simulink model "P2p2"  (R2014a)
settings: Solver=ode1  StartTime=0.0  StopTime=inf  FixedStep=0.002  RelTol=1e-3
PostLoadFcn:
  | qc_set_target_type(getConfigSet(bdroot, 'QUARC Default Target Configuration'));
values from neighbouring files (symbols this model uses):
  K_pd = -2*real(eig)*J_p/L1    [P2_init.m]
  K_pp = abs(eig)^2*J_p/L1    [P2_init.m]
  K_rp = -1.5    [P2_init.m]
undefined symbols (not defined in the file or in its folder): elevation_offset, HIL, Joystick_gain_x, Joystick_gain_y, qc_get_step_size, Vs_star_meas
libraries: simulink_extras x7, quarc_library x7
settings Model: SimulationMode=external  ExtModeTrigDuration=500000  Creator=Rchan  LastModifiedBy=rendellc
settings SolverCC: PositivePriorityOrder=on
settings DataIOCC: SignalLoggingSaveFormat=ModelDataLogs
settings OptimizationCC: ExpressionDepthLimit=2147483647  InitFltsAndDblsToZero=on
settings DebuggingCC: SaveWithParameterizedLinksMsg=none  UnderspecifiedInitializationDetection=Classic  MultiTaskDSMMsg=warning  MultiTaskCondExecSysMsg=none  FcnCallInpInsideContextMsg=UseLocalSettings  StateNameClashWarn=warning
settings RTWCC: SystemTargetFile=quarc_win64.tlc  TemplateMakefile=quarc_default_tmf  Description=QUARC Win64 Target  ProcessScript=quarc_win64_make_rtw_hook
settings STFCustomTargetCC: CPPClassGenCompliant=on
settings GRTTargetCC: ParMdlRefBuildCompliant=off  CompOptLevelCompliant=off  CombineOutputUpdateFcns=off  MatFileLogging=off  GRTInterface=on  ExtMode=on  ExtModeMexFile=quarc_comm

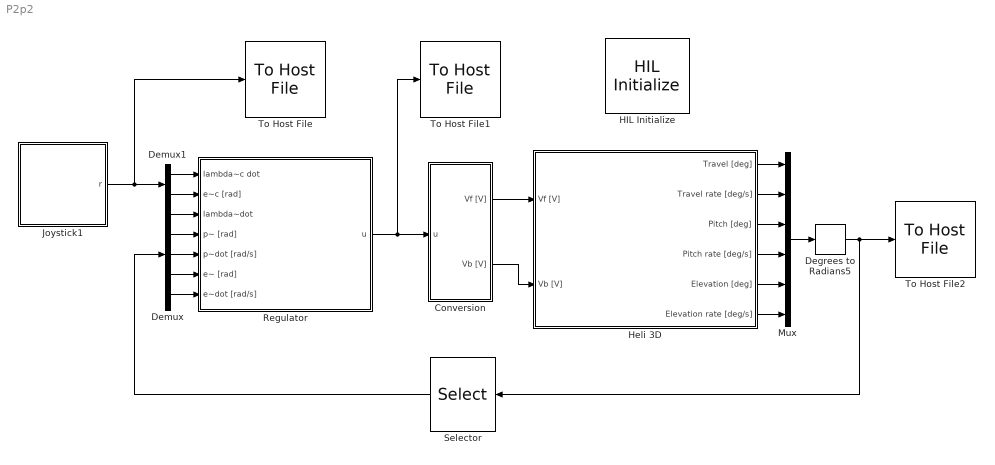
== system P2p2 ==
  Conversion : Subsystem
  Degrees to Radians5 : simulink_extras/Transformations/Degrees to Radians
  Demux : Demux  Outputs=5
  Demux1 : Demux  Outputs=2
  HIL Initialize : quarc_library/Data Acquisition/Generic/Configuration/HIL Initialize  Priority=-99  object_name=HIL-1  board_type=q8_usb  board_number=0  board_options=update_rate=normal;decimation=1  exclusive=off  active=off  hardware_clocks=[0:2]  clock_modes=[]  initial_clock_frequencies=[]  set_clock_params_at_start=off  set_clock_params_at_switch_in=off  set_clock_frequencies_at_start=off  set_clock_frequencies_at_switch_in=off  analog_input_channels=[0:7]  analog_input_maximums=10  analog_input_minimums=-10  set_analog_input_params_at_start=on  set_analog_input_params_at_switch_in=off  analog_output_channels=[0:7]  analog_output_maximums=10  analog_output_minimums=-10  initial_analog_outputs=[0]  final_analog_outputs=[0]  watchdog_analog_outputs=0  set_analog_output_params_at_start=on  set_analog_output_params_at_switch_in=off  set_analog_outputs_at_start=on  set_analog_outputs_at_switch_in=off  set_analog_outputs_at_terminate=on  set_analog_outputs_at_switch_out=off  set_analog_outputs_on_watchdog=off  digital_input_channels=[]  digital_output_channels=[]  digital_output_configuration=[]  initial_digital_outputs=[1]  final_digital_outputs=[1]  watchdog_digital_outputs=[1]  set_digital_output_params_at_start=off  set_digital_output_params_at_switch_in=off  set_digital_outputs_at_start=on  set_digital_outputs_at_switch_in=off  set_digital_outputs_at_terminate=on  set_digital_outputs_at_switch_out=off  set_digital_outputs_on_watchdog=off  encoder_channels=[0:7]  quadrature=[4]  encoder_filter_frequency=[]  initial_encoder_counts=[0]  set_encoder_params_at_start=on  set_encoder_params_at_switch_in=off  set_encoder_counts_at_start=on  set_encoder_counts_at_switch_in=off  pwm_channels=[0:7]  pwm_modes=0  pwm_frequency=99.532799999999995e6/4095  pwm_configuration=[0]  pwm_alignment=[0]  pwm_polarity=[1]  pwm_leading_deadband=[0]  pwm_trailing_deadband=[0]  initial_pwm_outputs=[0]  final_pwm_outputs=[0]  watchdog_pwm_outputs=[0]  set_pwm_params_at_start=on  set_pwm_params_at_switch_in=off  set_pwm_outputs_at_start=on  set_pwm_outputs_at_switch_in=off  set_pwm_outputs_at_terminate=on  set_pwm_outputs_at_switch_out=off  set_pwm_outputs_on_watchdog=off  other_output_channels=[]  initial_other_outputs=[]  final_other_outputs=[]  watchdog_other_outputs=[]  set_other_outputs_at_start=off  set_other_outputs_at_switch_in=off  set_other_outputs_at_terminate=off  set_other_outputs_at_switch_out=off  set_other_outputs_on_watchdog=off
  Heli 3D : Subsystem
  Joystick1 : Subsystem
      mask Display: image('../Common/joy_img.png');
  Mux : Mux  Inputs=6
  Regulator : Subsystem
  Selector : Selector  InputPortWidth=6  Indices=[2 3 4 5 6]
  To Host File : quarc_library/Sinks/To Host/To Host File  file_name=..\..\data\Part 2\P2p2_ref.mat  variable_name=ref  decimation=1  sample_time=-1  file_format=MAT-file v.4  options=No header or footer  append=off  final_file_name=..\..\data\Part 2\P2p2_ref.mat
  To Host File1 : quarc_library/Sinks/To Host/To Host File  file_name=P2p2_u.mat  variable_name=u  decimation=1  sample_time=-1  file_format=MAT-file v.4  options=No header or footer  append=off  final_file_name=P2p2_u.mat
  To Host File2 : quarc_library/Sinks/To Host/To Host File  file_name=P2p2_plant.mat  variable_name=plant  decimation=1  sample_time=-1  file_format=MAT-file v.4  options=No header or footer  append=off  final_file_name=P2p2_plant.mat
  wires:
  Conversion/2(Vb [V]) -> Heli 3D/2(Vb [V])
  Conversion/1(Vf [V]) -> Heli 3D/1(Vf [V])
  Heli 3D/1(Travel [deg]) -> Mux/1
  Heli 3D/2(Travel rate [deg/s]) -> Mux/2
  Heli 3D/3(Pitch [deg]) -> Mux/3
  Heli 3D/4(Pitch rate [deg/s]) -> Mux/4
  Heli 3D/6(Elevation rate [deg/s]) -> Mux/6
  Heli 3D/5(Elevation [deg]) -> Mux/5
  Mux/1 -> Degrees to Radians5/1
  Selector/1 -> Demux/1
  Demux/1 -> Regulator/3(lambda~dot)
  Demux/2 -> Regulator/4(p~ [rad])
  Demux/3 -> Regulator/5("p~dot [rad/s] ")
  Demux/4 -> Regulator/6(e~ [rad])
  Demux/5 -> Regulator/7(e~dot [rad/s])
  Demux1/1 -> Regulator/1(lambda~c dot)
  Demux1/2 -> Regulator/2(e~c [rad])
  Degrees to Radians5/1 -> To Host File2/1, Selector/1
  Joystick1/1(r) -> To Host File/1, Demux1/1
  Regulator/1(u) -> To Host File1/1, Conversion/1(u)

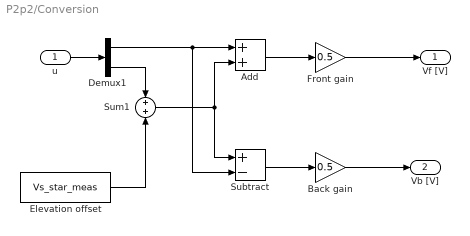
== system P2p2/Conversion ==
  u : Inport
  Add : Sum
  Back gain : Gain  Gain=0.5
  Demux1 : Demux  Outputs=2
  Elevation offset : Constant  Value=Vs_star_meas
  Front gain : Gain  Gain=0.5
  Subtract : Sum  Inputs=+-
  Sum1 : Sum  Inputs=+|+
  Vf [V] : Outport
  Vb [V] : Outport  Port=2
  wires:
  Demux1/1 -> Subtract/2, Add/1
  Subtract/1 -> Back gain/1
  Back gain/1 -> Vb [V]/1
  Add/1 -> Front gain/1
  Front gain/1 -> Vf [V]/1
  Elevation offset/1 -> Sum1/2
  Demux1/2 -> Sum1/1
  Sum1/1 -> Subtract/1, Add/2
  u/1 -> Demux1/1

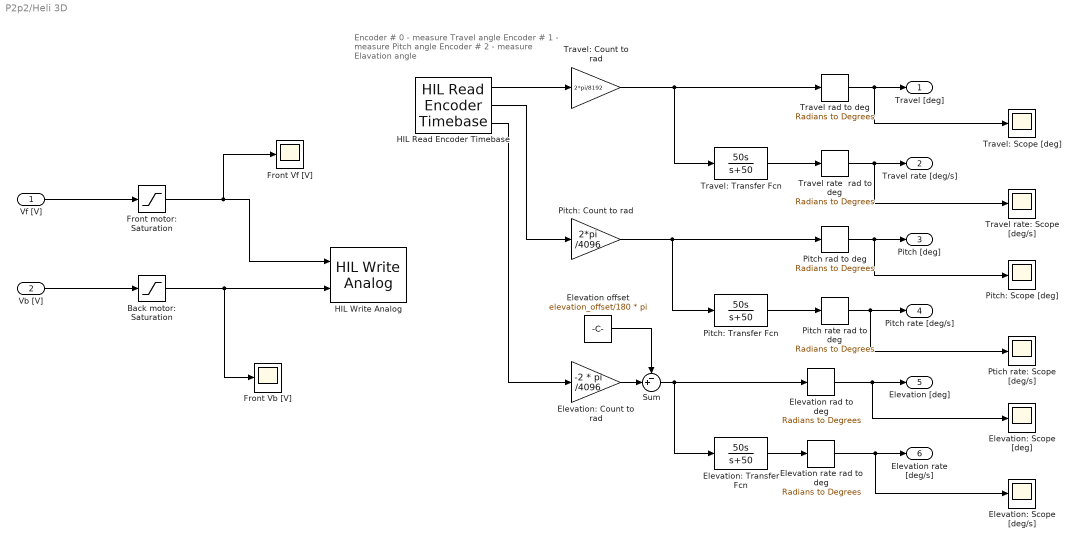
== system P2p2/Heli 3D ==
  note: Encoder # 0 - measure Travel angle
      | Encoder # 1 - measure Pitch angle
      | Encoder # 2 - measure Elavation angle
  Vf [V] : Inport
  Vb [V] : Inport  Port=2
  Back motor: Saturation : Saturate  UpperLimit=5  LowerLimit=-5
  Elevation offset : Constant  Value=elevation_offset/180 * pi
  Elevation rad to deg : simulink_extras/Transformations/Radians to Degrees
  Elevation rate rad to deg : simulink_extras/Transformations/Radians to Degrees
  Elevation: Count to rad : Gain  Gain=-2 * pi /4096
  Elevation: Scope [deg/s] : Scope
      settings: YMin=-15  YMax=15  SaveName=ScopeData13
  Elevation: Scope [deg] : Scope
      settings: YMax=45  SaveName=ScopeData12
  Elevation: Transfer Fcn : TransferFcn  Numerator=[50 0]  Denominator=[1 50]
  Front Vb [V] : Scope
      settings: YMin=-2  SaveName=ScopeData2
  Front Vf [V] : Scope
      settings: YMin=-2
  Front motor: Saturation : Saturate  UpperLimit=5  LowerLimit=-5
  HIL Read Encoder Timebase : quarc_library/Data Acquisition/Generic/Timebases/HIL Read Encoder Timebase  object_name=HIL-1  clock=0  channels=[0:2]  samples_in_buffer=max(ceil(1/qc_get_step_size), 1)  active=on  vector_output=off  data_type_mode=Inherit via back propagation  data_type=double
  HIL Write Analog : quarc_library/Data Acquisition/Generic/Immediate I//O/HIL Write Analog  object_name=HIL-1  channels=[0:1]  sample_time=-1  active=off  vector_input=off
  Pitch rad to deg : simulink_extras/Transformations/Radians to Degrees
  Pitch rate rad to deg : simulink_extras/Transformations/Radians to Degrees
  Pitch: Count to rad : Gain  Gain=2*pi /4096
  Pitch: Scope [deg] : Scope
      settings: YMin=-80  YMax=80  SaveName=ScopeData10
  Pitch: Transfer Fcn : TransferFcn  Numerator=[50 0]  Denominator=[1 50]
  Ptich rate: Scope [deg/s] : Scope
      settings: YMin=-15  YMax=15  SaveName=ScopeData11
  Sum : Sum  Inputs=-+|
  Travel rad to deg : simulink_extras/Transformations/Radians to Degrees
  Travel rate  rad to deg : simulink_extras/Transformations/Radians to Degrees
  Travel rate: Scope [deg/s] : Scope
      settings: YMin=-30  YMax=70  SaveName=ScopeData9
  Travel: Count to rad : Gain  Gain=2*pi/8192
  Travel: Scope [deg] : Scope
      settings: YMin=-250  YMax=2250  SaveName=ScopeData8
  Travel: Transfer Fcn : TransferFcn  Numerator=[50 0]  Denominator=[1 50]
  Travel [deg] : Outport
  Travel rate [deg/s] : Outport  Port=2
  Pitch [deg] : Outport  Port=3
  Pitch rate [deg/s] : Outport  Port=4
  Elevation [deg] : Outport  Port=5
  Elevation rate [deg/s] : Outport  Port=6
  wires:
  HIL Read Encoder Timebase/1 -> Travel: Count to rad/1
  HIL Read Encoder Timebase/2 -> Pitch: Count to rad/1
  HIL Read Encoder Timebase/3 -> Elevation: Count to rad/1
  Travel: Count to rad/1 -> Travel: Transfer Fcn/1, Travel rad to deg/1
  Travel: Transfer Fcn/1 -> Travel rate  rad to deg/1
  Pitch: Count to rad/1 -> Pitch: Transfer Fcn/1, Pitch rad to deg/1
  Pitch: Transfer Fcn/1 -> Pitch rate rad to deg/1
  Elevation: Transfer Fcn/1 -> Elevation rate rad to deg/1
  Travel rad to deg/1 -> Travel: Scope [deg]/1, Travel [deg]/1
  Travel rate  rad to deg/1 -> Travel rate: Scope [deg/s]/1, Travel rate [deg/s]/1
  Pitch rad to deg/1 -> Pitch: Scope [deg]/1, Pitch [deg]/1
  Pitch rate rad to deg/1 -> Ptich rate: Scope [deg/s]/1, Pitch rate [deg/s]/1
  Elevation rad to deg/1 -> Elevation: Scope [deg]/1, Elevation [deg]/1
  Elevation rate rad to deg/1 -> Elevation: Scope [deg/s]/1, Elevation rate [deg/s]/1
  Vf [V]/1 -> Front motor: Saturation/1
  Vb [V]/1 -> Back motor: Saturation/1
  Back motor: Saturation/1 -> Front Vb [V]/1, HIL Write Analog/2
  Elevation: Count to rad/1 -> Sum/2
  Sum/1 -> Elevation: Transfer Fcn/1, Elevation rad to deg/1
  Elevation offset/1 -> Sum/1
  Front motor: Saturation/1 -> Front Vf [V]/1, HIL Write Analog/1

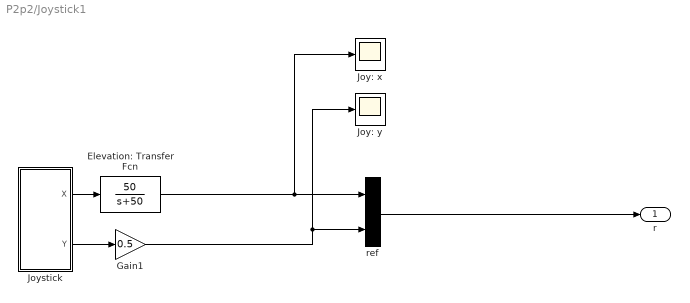
== system P2p2/Joystick1 ==
  Elevation: Transfer Fcn : TransferFcn  Numerator=[0 50]  Denominator=[1 50]
  Gain1 : Gain  Gain=0.5
  Joy: x : Scope
  Joy: y : Scope
      settings: SaveName=ScopeData3
  Joystick : Subsystem
  ref : Concatenate
  r : Outport
  wires:
  Elevation: Transfer Fcn/1 -> Joy: x/1, ref/1
  Joystick/2(Y) -> Gain1/1
  ref/1 -> r/1
  Gain1/1 -> Joy: y/1, ref/2
  Joystick/1(X) -> Elevation: Transfer Fcn/1

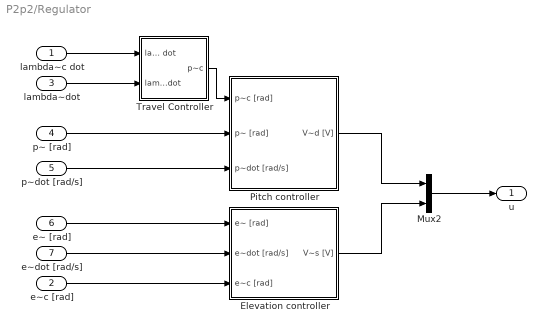
== system P2p2/Regulator ==
  lambda~c dot : Inport
  e~c [rad] : Inport  Port=2
  lambda~dot : Inport  Port=3
  p~ [rad] : Inport  Port=4
  "p~dot [rad/s] " : Inport  Port=5
  e~ [rad] : Inport  Port=6
  e~dot [rad/s] : Inport  Port=7
  Elevation controller : Subsystem
  Mux2 : Mux  Inputs=2
  Pitch controller : Subsystem
  "Travel Controller " : Subsystem
  u : Outport
  wires:
  lambda~dot/1 -> "Travel Controller "/2(lamba~dot)
  "p~dot [rad/s] "/1 -> Pitch controller/3(p~dot [rad/s])
  e~c [rad]/1 -> Elevation controller/3(e~c [rad])
  p~ [rad]/1 -> Pitch controller/2(p~ [rad])
  lambda~c dot/1 -> "Travel Controller "/1(lamba~c dot)
  e~dot [rad/s]/1 -> Elevation controller/2(e~dot [rad/s])
  e~ [rad]/1 -> Elevation controller/1(e~ [rad])
  "Travel Controller "/1(p~c) -> Pitch controller/1(p~c [rad])
  Pitch controller/1(V~d [V]) -> Mux2/1
  Elevation controller/1(V~s [V]) -> Mux2/2
  Mux2/1 -> u/1

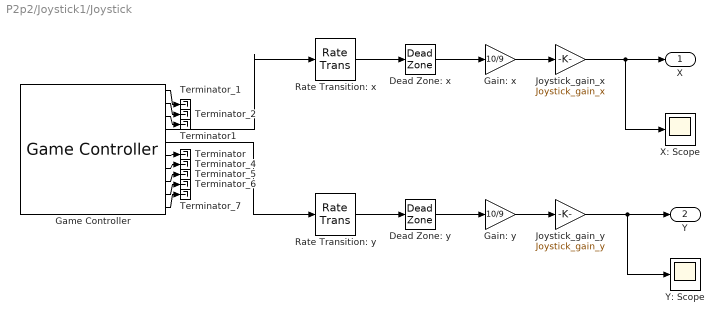
== system P2p2/Joystick1/Joystick ==
  Dead Zone: x : DeadZone  LowerValue=-0.1  UpperValue=0.1  SaturateOnIntegerOverflow=on
  Dead Zone: y : DeadZone  LowerValue=-0.1  UpperValue=0.1  SaturateOnIntegerOverflow=on
  Gain: x : Gain  Gain=10/9
  Gain: y : Gain  Gain=10/9
  Game Controller : quarc_library/Devices/Peripherals/Target/Game Controller  controller=1  buffer_size=12  deadzone=[]  saturation=[]  sample_time=max(qc_get_step_size, 0.01)  auto_center=off  enabled=on
  Joystick_gain_x : Gain  Gain=Joystick_gain_x
  Joystick_gain_y : Gain  Gain=Joystick_gain_y
  Rate Transition: x : RateTransition
  Rate Transition: y : RateTransition
  Terminator : Terminator
  Terminator1 : Terminator
  Terminator_{1..2,4..7} (6 alike) : Terminator
  X: Scope : Scope
      settings: YMin=-1  YMax=1  SaveName=ScopeData7
  Y: Scope : Scope
      settings: YMin=-10  YMax=10  SaveName=ScopeData5
  X : Outport
  Y : Outport  Port=2
  wires:
  Rate Transition: y/1 -> Dead Zone: y/1
  Rate Transition: x/1 -> Dead Zone: x/1
  Game Controller/5 -> Rate Transition: y/1
  Game Controller/4 -> Rate Transition: x/1
  Game Controller/1 -> Terminator_1/1
  Game Controller/2 -> Terminator_2/1
  Game Controller/7 -> Terminator_4/1
  Game Controller/8 -> Terminator_5/1
  Game Controller/9 -> Terminator_6/1
  Game Controller/10 -> Terminator_7/1
  Game Controller/3 -> Terminator1/1
  Game Controller/6 -> Terminator/1
  Dead Zone: x/1 -> Gain: x/1
  Dead Zone: y/1 -> Gain: y/1
  Gain: x/1 -> Joystick_gain_x/1
  Gain: y/1 -> Joystick_gain_y/1
  Joystick_gain_x/1 -> X/1, X: Scope/1
  Joystick_gain_y/1 -> Y: Scope/1, Y/1

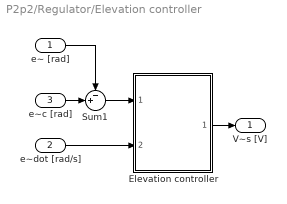
== system P2p2/Regulator/Elevation controller ==
  e~ [rad] : Inport
  e~dot [rad/s] : Inport  Port=2
  e~c [rad] : Inport  Port=3
  Elevation controller : Subsystem
  Sum1 : Sum  Inputs=-+|
  V~s [V] : Outport  InitialOutput=0
  wires:
  Sum1/1 -> Elevation controller/1(e~ [rad])
  Elevation controller/1(V~_s [V]) -> V~s [V]/1
  e~ [rad]/1 -> Sum1/1
  e~dot [rad/s]/1 -> Elevation controller/2(e~_dot [rad/s])
  e~c [rad]/1 -> Sum1/2

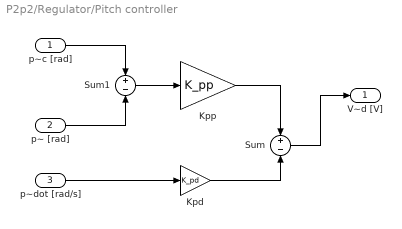
== system P2p2/Regulator/Pitch controller ==
  p~c [rad] : Inport
  p~ [rad] : Inport  Port=2
  p~dot [rad/s] : Inport  Port=3
  Kpd : Gain  Gain=K_pd
  "Kpp " : Gain  Gain=K_pp
  Sum : Sum  Inputs=+|-
  Sum1 : Sum  Inputs=+|-
  V~d [V] : Outport  InitialOutput=0
  wires:
  p~c [rad]/1 -> Sum1/1
  p~ [rad]/1 -> Sum1/2
  Sum1/1 -> "Kpp "/1
  "Kpp "/1 -> Sum/1
  Kpd/1 -> Sum/2
  p~dot [rad/s]/1 -> Kpd/1
  Sum/1 -> V~d [V]/1

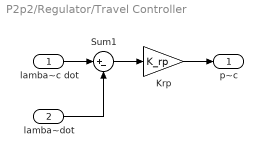
== system P2p2/Regulator/Travel Controller  ==
  lamba~c dot : Inport
  lamba~dot : Inport  Port=2
  Krp : Gain  Gain=K_rp
  Sum1 : Sum  Inputs=|+-
  p~c : Outport
  wires:
  Krp/1 -> p~c/1
  lamba~c dot/1 -> Sum1/1
  lamba~dot/1 -> Sum1/2
  Sum1/1 -> Krp/1

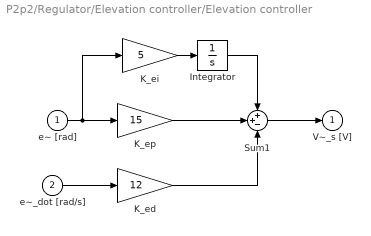
== system P2p2/Regulator/Elevation controller/Elevation controller ==
  e~ [rad] : Inport
  e~_dot [rad/s] : Inport  Port=2
  Integrator : Integrator  LimitOutput=on
  K_ed : Gain  Gain=12  SaturateOnIntegerOverflow=on  OutDataTypeStr=Inherit: Same as input  ParamDataTypeStr=Inherit: Same as input
  K_ei : Gain  Gain=5  SaturateOnIntegerOverflow=on  OutDataTypeStr=Inherit: Same as input  ParamDataTypeStr=Inherit: Same as input
  K_ep : Gain  Gain=15  SaturateOnIntegerOverflow=on  OutDataTypeStr=Inherit: Same as input  ParamDataTypeStr=Inherit: Same as input
  Sum1 : Sum  Inputs=++-
  V~_s [V] : Outport  InitialOutput=0
  wires:
  K_ei/1 -> Integrator/1
  Integrator/1 -> Sum1/1
  Sum1/1 -> V~_s [V]/1
  e~_dot [rad/s]/1 -> K_ed/1
  K_ed/1 -> Sum1/3
  K_ep/1 -> Sum1/2
  e~ [rad]/1 -> K_ep/1, K_ei/1
